simulink model "meat_1024pt_bee2_fpv2"  (Simulink 6.2)
settings: Solver=ode45  StartTime=0.0  StopTime=60000  RelTol=1e-3
undefined symbols (not defined in the file): BEE2_usr, bit_rev, pfb_coeff_gen_calc
libraries: xbsIndex_r3 x1085, casper_library x94, xps_library x27
(part 5 of 8)

== system meat_1024pt_bee2_fpv2/fft/fft_biplex0/biplex_core/fft_stage_1 ==
  in1 : Inport  Port=1  LatchInput=off
  in2 : Inport  Port=2  LatchInput=off
  sync : Inport  Port=3  LatchInput=off
  shift : Inport  Port=4  LatchInput=off
  Counter : xbsIndex_r3/Counter  cnt_type=Free Running  n_bits=FFTSize-FFTStage+1  bin_pt=0  arith_type=Unsigned  start_count=0  cnt_to=Inf  cnt_by_val=1  operation=Up  explicit_period=off  period=1  load_pin=off  rst=on  en=off  dbl_ovrd=off  show_param=off  use_rpm=off  gen_core=on
      settings: xl_area=[0, 0, 0, 0, 0, 0, 0]
  Delay : xbsIndex_r3/Delay  latency=1  reg_retiming=off  explicit_period=off  period=1  en=off  accept_only_valid=off  init_zero=on  dbl_ovrd=off  show_param=off
      settings: xl_area=[0, 0, 0, 0, 0, 0, 0]
  Mux : xbsIndex_r3/Mux  inputs=2  precision=Full  arith_type="Signed  (2's comp)"  n_bits=8  bin_pt=2  quantization=Truncate  overflow=Wrap  latency=1  explicit_period=off  period=1  en=off  dbl_ovrd=off  show_param=off  mux_type=off  use_rpm=off  gen_core=on
      settings: xl_area=[0, 0, 0, 0, 0, 0, 0]
  Mux1 : xbsIndex_r3/Mux  inputs=2  precision=Full  arith_type="Signed  (2's comp)"  n_bits=8  bin_pt=2  quantization=Truncate  overflow=Wrap  latency=1  explicit_period=off  period=1  en=off  dbl_ovrd=off  show_param=off  mux_type=off  use_rpm=off  gen_core=on
      settings: xl_area=[0, 0, 0, 0, 0, 0, 0]
  Slice : xbsIndex_r3/Slice  Orientation=up  mode=Lower Bit Location + Width  nbits=1  bit1=-(FFTStage - 1)  base1=MSB of Input  bit0=FFTStage - 1  base0=LSB of Input  boolean_output=on  explicit_period=off  period=1  dbl_ovrd=off
  Slice1 : xbsIndex_r3/Slice  mode=Upper Bit Location + Width  nbits=1  bit1=0  base1=MSB of Input  bit0=0  base0=LSB of Input  boolean_output=off  explicit_period=off  period=1  dbl_ovrd=off
  butterfly : Subsystem
  delay_b : Subsystem  BlockChoice=delay_bram
      link override delay_bram: bram_latency=bram_latency  DelayLen=2^(FFTSize-FFTStage)
      link override delay_bram/Constant2: equ=P=C
      link override delay_slr: DelayLen=2^(FFTSize-FFTStage)
      settings: AttributesFormatString=%<BlockChoice>  TemplateBlock=casper_library/Delays/delay  MemberBlocks=delay_bram,delay_slr
  delay_f : Subsystem  BlockChoice=delay_bram
      link override delay_bram: bram_latency=bram_latency  DelayLen=2^(FFTSize-FFTStage)
      link override delay_bram/Constant2: equ=P=C
      link override delay_slr: DelayLen=2^(FFTSize-FFTStage)
      settings: AttributesFormatString=%<BlockChoice>  TemplateBlock=casper_library/Delays/delay  MemberBlocks=delay_bram,delay_slr
  sync_delay : casper_library/Delays/sync_delay  DelayLen=2^(FFTSize - FFTStage)
      link override Constant: equ=P=C
      link override Constant1: equ=P=C
      link override Constant2: equ=P=C
      link override Constant3: equ=P=C
  out1 : Outport
  out2 : Outport  Port=2
  of : Outport  Port=3
  sync_out : Outport  Port=4
  wires:
  shift/1 -> Slice/1
  Delay/1 -> sync_delay/1
  sync/1 -> Counter/1, Delay/1
  Counter/1 -> Slice1/1
  Mux/1 -> butterfly/2(b)
  Mux1/1 -> delay_b/1(In1)
  delay_f/1(Out1) -> Mux1/3, Mux/2
  in1/1 -> Mux/3, Mux1/2
  Slice1/1 -> Mux/1, Mux1/1
  in2/1 -> delay_f/1(In1)
  delay_b/1(Out1) -> butterfly/1(a)
  sync_delay/1 -> butterfly/3(sync)
  Slice/1 -> butterfly/4(shift)
  butterfly/3(of) -> of/1
  butterfly/2(a-bw) -> out2/1
  butterfly/1(a+bw) -> out1/1
  butterfly/4(sync_out) -> sync_out/1

== system meat_1024pt_bee2_fpv2/fft/fft_biplex0/biplex_core/fft_stage_10 ==
  in1 : Inport  Port=1  LatchInput=off
  in2 : Inport  Port=2  LatchInput=off
  of_in : Inport  Port=3  LatchInput=off
  sync : Inport  Port=4  LatchInput=off
  shift : Inport  Port=5  LatchInput=off
  Counter : xbsIndex_r3/Counter  cnt_type=Free Running  n_bits=FFTSize-FFTStage+1  bin_pt=0  arith_type=Unsigned  start_count=0  cnt_to=Inf  cnt_by_val=1  operation=Up  explicit_period=off  period=1  load_pin=off  rst=on  en=off  dbl_ovrd=off  show_param=off  use_rpm=off  gen_core=on
      settings: xl_area=[0, 0, 0, 0, 0, 0, 0]
  Delay : xbsIndex_r3/Delay  latency=1  reg_retiming=off  explicit_period=off  period=1  en=off  accept_only_valid=off  init_zero=on  dbl_ovrd=off  show_param=off
      settings: xl_area=[0, 0, 0, 0, 0, 0, 0]
  Logical1 : xbsIndex_r3/Logical  logical_function=OR  inputs=2  precision=Full  arith_type=Unsigned  n_bits=8  bin_pt=2  align_bp=on  latency=1  explicit_period=on  period=1  en=off  dbl_ovrd=off  show_param=off
      settings: xl_area=[0, 0, 0, 0, 0, 0, 0]
  Mux : xbsIndex_r3/Mux  inputs=2  precision=Full  arith_type="Signed  (2's comp)"  n_bits=8  bin_pt=2  quantization=Truncate  overflow=Wrap  latency=1  explicit_period=off  period=1  en=off  dbl_ovrd=off  show_param=off  mux_type=off  use_rpm=off  gen_core=on
      settings: xl_area=[0, 0, 0, 0, 0, 0, 0]
  Mux1 : xbsIndex_r3/Mux  inputs=2  precision=Full  arith_type="Signed  (2's comp)"  n_bits=8  bin_pt=2  quantization=Truncate  overflow=Wrap  latency=1  explicit_period=off  period=1  en=off  dbl_ovrd=off  show_param=off  mux_type=off  use_rpm=off  gen_core=on
      settings: xl_area=[0, 0, 0, 0, 0, 0, 0]
  Slice : xbsIndex_r3/Slice  Orientation=up  mode=Lower Bit Location + Width  nbits=1  bit1=-(FFTStage - 1)  base1=MSB of Input  bit0=FFTStage - 1  base0=LSB of Input  boolean_output=on  explicit_period=off  period=1  dbl_ovrd=off
  Slice1 : xbsIndex_r3/Slice  mode=Upper Bit Location + Width  nbits=1  bit1=0  base1=MSB of Input  bit0=0  base0=LSB of Input  boolean_output=off  explicit_period=off  period=1  dbl_ovrd=off
  butterfly_direct : Subsystem  AncestorBlock=casper_library/FFTs/butterfly_direct  mask(butterfly_direct){FFTSize=10, Coeffs=getfield( getfield( get_param( gcb,'UserData'), 'parameters'),'Coeffs'), StepPeriod=0, BitWidth=18, add_latency=3, mult_latency=4, bram_latency=3, use_bram=0, quantization=Truncate, overflow=Wrap}
      mask prompts: FFTSize "Size of FFT: (2^?)"; Coeffs "Coefficients: (0 to 2^(FFTSize-1)-1)"; StepPeriod "Coefficient Step Period: (2^?)"; BitWidth "Output Bitwidth:"; add_latency "Add Latency"; mult_latency "Mult Latency"; bram_latency "BRAM Latency"; use_bram "Store Coefficients in BRAM"; quantization "Quantization Behavior"; overflow "Overflow Behavior"
      mask init:
      | butterfly_direct_init(gcb,...
      |               'FFTSize', FFTSize,...
      |               'Coeffs', Coeffs,...
      |               'StepPeriod', StepPeriod,...
      |               'BitWidth', BitWidth,...
      |               'add_latency', add_latency,...
      |               'mult_latency', mult_latency,...
      |               'bram_latency', bram_latency,...
      |               'use_bram',use_bram,...
      |               'quantization',quantization,...
      |               'overflow',overflow);
      settings: AttributesFormatString=|
      | FFTSize=10, Coeffs=[0    1    2    3    4    5    6    7    8    9   10   11   12   13   14   15   16   17   18   19   20   21   22   23   24   25   26   27   28   29   30   31   32   33   34   35   36   37   38   39   40   41   42   43   44   45   46   47   48   49   50   51   52   53   54   55   56   57   58   59   60   61   62   63   64   65   66   67   68   69   70   71   72   73   74   75   76   77   78   79   80   81   82   83   84   85   86   87   88   89   90   91   92   93   94   95   96   97   98   99  100  101  102  103  104  105  106  107  108  109  110  111  112  113  114  115  116  117  118  119  120  121  122  123  124  125  126  127  128  129  130  131  132  133  134  135  136  137  138  139  140  141  142  143  144  145  146  147  148  149  150  151  152  153  154  155  156  157  158  159  160  161  162  163  164  165  166  167  168  169  170  171  172  173  174  175  176  177  178  179  180  181  182  183  184  185  186  187  188  189  190  191  192  193  194  195  196  197  198  199  200  201  202  203  204  205  206  207  208  209  210  211  212  213  214  215  216  217  218  219  220  221  222  223  224  225  226  227  228  229  230  231  232  233  234  235  236  237  238  239  240  241  242  243  244  245  246  247  248  249  250  251  252  253  254  255  256  257  258  259  260  261  262  263  264  265  266  267  268  269  270  271  272  273  274  275  276  277  278  279  280  281  282  283  284  285  286  287  288  289  290  291  292  293  294  295  296  297  298  299  300  301  302  303  304  305  306  307  308  309  310  311  312  313  314  315  316  317  318  319  320  321  322  323  324  325  326  327  328  329  330  331  332  333  334  335  336  337  338  339  340  341  342  343  344  345  346  347  348  349  350  351  352  353  354  355  356  357  358  359  360  361  362  363  364  365  366  367  368  369  370  371  372  373  374  375  376  377  378  379  380  381  382  383  384  385  386  387  388  389  390  391  392  393  394  395  396  397  398  399  400  401  402  403  404  405  406  407  408  409  410  411  412  413  414  415  416  417  418  419  420  421  422  423  424  425  426  427  428  429  430  431  432  433  434  435  436  437  438  439  440  441  442  443  444  445  446  447  448  449  450  451  452  453  454  455  456  457  458  459  460  461  462  463  464  465  466  467  468  469  470  471  472  473  474  475  476  477  478  479  480  481  482  483  484  485  486  487  488  489  490  491  492  493  494  495  496  497  498  499  500  501  502  503  504  505  506  507  508  509  510  511],
      |  StepPeriod=0, BitWidth=18
      mask StyleString: edit,edit,edit,edit,edit,edit,edit,edit,popup(Truncate|Round  (unbiased: +/- Inf)|Round  (unbiased: Even Values)),popup(Wrap|Saturate|Error)
  delay_b : Subsystem  BlockChoice=delay_slr
      link override delay_bram: bram_latency=bram_latency  DelayLen=2^(FFTSize-FFTStage)
      link override delay_slr: DelayLen=2^(FFTSize-FFTStage)
      settings: AttributesFormatString=%<BlockChoice>  TemplateBlock=casper_library/Delays/delay  MemberBlocks=delay_bram,delay_slr
  delay_f : Subsystem  BlockChoice=delay_slr
      link override delay_bram: bram_latency=bram_latency  DelayLen=2^(FFTSize-FFTStage)
      link override delay_slr: DelayLen=2^(FFTSize-FFTStage)
      settings: AttributesFormatString=%<BlockChoice>  TemplateBlock=casper_library/Delays/delay  MemberBlocks=delay_bram,delay_slr
  sync_delay : casper_library/Delays/sync_delay  DelayLen=2^(FFTSize - FFTStage)
      link override Constant: equ=P=C
      link override Constant1: equ=P=C
      link override Constant2: equ=P=C
      link override Constant3: equ=P=C
  out1 : Outport
  out2 : Outport  Port=2
  of : Outport  Port=3
  sync_out : Outport  Port=4
  wires:
  butterfly_direct/4(sync_out) -> sync_out/1
  butterfly_direct/1(a+bw) -> out1/1
  butterfly_direct/2(a-bw) -> out2/1
  butterfly_direct/3(of) -> Logical1/1
  Slice/1 -> butterfly_direct/4(shift)
  sync_delay/1 -> butterfly_direct/3(sync)
  delay_b/1(Out1) -> butterfly_direct/1(a)
  in2/1 -> delay_f/1(In1)
  Slice1/1 -> Mux1/1, Mux/1
  in1/1 -> Mux1/2, Mux/3
  delay_f/1(Out1) -> Mux/2, Mux1/3
  Mux1/1 -> delay_b/1(In1)
  Mux/1 -> butterfly_direct/2(b)
  Counter/1 -> Slice1/1
  sync/1 -> Delay/1, Counter/1
  Delay/1 -> sync_delay/1
  Logical1/1 -> of/1
  of_in/1 -> Logical1/2
  shift/1 -> Slice/1

== system meat_1024pt_bee2_fpv2/fft/fft_biplex0/biplex_core/fft_stage_2 ==
  in1 : Inport  Port=1  LatchInput=off
  in2 : Inport  Port=2  LatchInput=off
  of_in : Inport  Port=3  LatchInput=off
  sync : Inport  Port=4  LatchInput=off
  shift : Inport  Port=5  LatchInput=off
  Counter : xbsIndex_r3/Counter  cnt_type=Free Running  n_bits=FFTSize-FFTStage+1  bin_pt=0  arith_type=Unsigned  start_count=0  cnt_to=Inf  cnt_by_val=1  operation=Up  explicit_period=off  period=1  load_pin=off  rst=on  en=off  dbl_ovrd=off  show_param=off  use_rpm=off  gen_core=on
      settings: xl_area=[0, 0, 0, 0, 0, 0, 0]
  Delay : xbsIndex_r3/Delay  latency=1  reg_retiming=off  explicit_period=off  period=1  en=off  accept_only_valid=off  init_zero=on  dbl_ovrd=off  show_param=off
      settings: xl_area=[0, 0, 0, 0, 0, 0, 0]
  Logical1 : xbsIndex_r3/Logical  logical_function=OR  inputs=2  precision=Full  arith_type=Unsigned  n_bits=8  bin_pt=2  align_bp=on  latency=1  explicit_period=on  period=1  en=off  dbl_ovrd=off  show_param=off
      settings: xl_area=[0, 0, 0, 0, 0, 0, 0]
  Mux : xbsIndex_r3/Mux  inputs=2  precision=Full  arith_type="Signed  (2's comp)"  n_bits=8  bin_pt=2  quantization=Truncate  overflow=Wrap  latency=1  explicit_period=off  period=1  en=off  dbl_ovrd=off  show_param=off  mux_type=off  use_rpm=off  gen_core=on
      settings: xl_area=[0, 0, 0, 0, 0, 0, 0]
  Mux1 : xbsIndex_r3/Mux  inputs=2  precision=Full  arith_type="Signed  (2's comp)"  n_bits=8  bin_pt=2  quantization=Truncate  overflow=Wrap  latency=1  explicit_period=off  period=1  en=off  dbl_ovrd=off  show_param=off  mux_type=off  use_rpm=off  gen_core=on
      settings: xl_area=[0, 0, 0, 0, 0, 0, 0]
  Slice : xbsIndex_r3/Slice  Orientation=up  mode=Lower Bit Location + Width  nbits=1  bit1=-(FFTStage - 1)  base1=MSB of Input  bit0=FFTStage - 1  base0=LSB of Input  boolean_output=on  explicit_period=off  period=1  dbl_ovrd=off
  Slice1 : xbsIndex_r3/Slice  mode=Upper Bit Location + Width  nbits=1  bit1=0  base1=MSB of Input  bit0=0  base0=LSB of Input  boolean_output=off  explicit_period=off  period=1  dbl_ovrd=off
  butterfly_direct : Subsystem  AncestorBlock=casper_library/FFTs/butterfly_direct  mask(butterfly_direct){FFTSize=10, Coeffs=[0 1], StepPeriod=8, BitWidth=18, add_latency=3, mult_latency=4, bram_latency=3, use_bram=1, quantization=Truncate, overflow=Wrap}
      mask prompts: FFTSize "Size of FFT: (2^?)"; Coeffs "Coefficients: (0 to 2^(FFTSize-1)-1)"; StepPeriod "Coefficient Step Period: (2^?)"; BitWidth "Output Bitwidth:"; add_latency "Add Latency"; mult_latency "Mult Latency"; bram_latency "BRAM Latency"; use_bram "Store Coefficients in BRAM"; quantization "Quantization Behavior"; overflow "Overflow Behavior"
      mask init: same as meat_1024pt_bee2_fpv2/fft/fft_biplex0/biplex_core/fft_stage_10/butterfly_direct
      settings: AttributesFormatString=|
      | FFTSize=10, Coeffs=[0  1],
      |  StepPeriod=8, BitWidth=18
      mask StyleString: edit,edit,edit,edit,edit,edit,edit,edit,popup(Truncate|Round  (unbiased: +/- Inf)|Round  (unbiased: Even Values)),popup(Wrap|Saturate|Error)
  delay_b : Subsystem  BlockChoice=delay_bram
      link override delay_bram: bram_latency=bram_latency  DelayLen=2^(FFTSize-FFTStage)
      link override delay_bram/Constant2: equ=P=C
      link override delay_slr: DelayLen=2^(FFTSize-FFTStage)
      settings: AttributesFormatString=%<BlockChoice>  TemplateBlock=casper_library/Delays/delay  MemberBlocks=delay_bram,delay_slr
  delay_f : Subsystem  BlockChoice=delay_bram
      link override delay_bram: bram_latency=bram_latency  DelayLen=2^(FFTSize-FFTStage)
      link override delay_bram/Constant2: equ=P=C
      link override delay_slr: DelayLen=2^(FFTSize-FFTStage)
      settings: AttributesFormatString=%<BlockChoice>  TemplateBlock=casper_library/Delays/delay  MemberBlocks=delay_bram,delay_slr
  sync_delay : casper_library/Delays/sync_delay  DelayLen=2^(FFTSize - FFTStage)
      link override Constant: equ=P=C
      link override Constant1: equ=P=C
      link override Constant2: equ=P=C
      link override Constant3: equ=P=C
  out1 : Outport
  out2 : Outport  Port=2
  of : Outport  Port=3
  sync_out : Outport  Port=4
  wires:
  butterfly_direct/4(sync_out) -> sync_out/1
  butterfly_direct/1(a+bw) -> out1/1
  butterfly_direct/2(a-bw) -> out2/1
  butterfly_direct/3(of) -> Logical1/1
  Slice/1 -> butterfly_direct/4(shift)
  sync_delay/1 -> butterfly_direct/3(sync)
  delay_b/1(Out1) -> butterfly_direct/1(a)
  in2/1 -> delay_f/1(In1)
  Slice1/1 -> Mux1/1, Mux/1
  in1/1 -> Mux1/2, Mux/3
  delay_f/1(Out1) -> Mux/2, Mux1/3
  Mux1/1 -> delay_b/1(In1)
  Mux/1 -> butterfly_direct/2(b)
  Counter/1 -> Slice1/1
  sync/1 -> Delay/1, Counter/1
  Delay/1 -> sync_delay/1
  Logical1/1 -> of/1
  of_in/1 -> Logical1/2
  shift/1 -> Slice/1

== system meat_1024pt_bee2_fpv2/fft/fft_biplex0/biplex_core/fft_stage_3 ==
  in1 : Inport  Port=1  LatchInput=off
  in2 : Inport  Port=2  LatchInput=off
  of_in : Inport  Port=3  LatchInput=off
  sync : Inport  Port=4  LatchInput=off
  shift : Inport  Port=5  LatchInput=off
  Counter : xbsIndex_r3/Counter  cnt_type=Free Running  n_bits=FFTSize-FFTStage+1  bin_pt=0  arith_type=Unsigned  start_count=0  cnt_to=Inf  cnt_by_val=1  operation=Up  explicit_period=off  period=1  load_pin=off  rst=on  en=off  dbl_ovrd=off  show_param=off  use_rpm=off  gen_core=on
      settings: xl_area=[0, 0, 0, 0, 0, 0, 0]
  Delay : xbsIndex_r3/Delay  latency=1  reg_retiming=off  explicit_period=off  period=1  en=off  accept_only_valid=off  init_zero=on  dbl_ovrd=off  show_param=off
      settings: xl_area=[0, 0, 0, 0, 0, 0, 0]
  Logical1 : xbsIndex_r3/Logical  logical_function=OR  inputs=2  precision=Full  arith_type=Unsigned  n_bits=8  bin_pt=2  align_bp=on  latency=1  explicit_period=on  period=1  en=off  dbl_ovrd=off  show_param=off
      settings: xl_area=[0, 0, 0, 0, 0, 0, 0]
  Mux : xbsIndex_r3/Mux  inputs=2  precision=Full  arith_type="Signed  (2's comp)"  n_bits=8  bin_pt=2  quantization=Truncate  overflow=Wrap  latency=1  explicit_period=off  period=1  en=off  dbl_ovrd=off  show_param=off  mux_type=off  use_rpm=off  gen_core=on
      settings: xl_area=[0, 0, 0, 0, 0, 0, 0]
  Mux1 : xbsIndex_r3/Mux  inputs=2  precision=Full  arith_type="Signed  (2's comp)"  n_bits=8  bin_pt=2  quantization=Truncate  overflow=Wrap  latency=1  explicit_period=off  period=1  en=off  dbl_ovrd=off  show_param=off  mux_type=off  use_rpm=off  gen_core=on
      settings: xl_area=[0, 0, 0, 0, 0, 0, 0]
  Slice : xbsIndex_r3/Slice  Orientation=up  mode=Lower Bit Location + Width  nbits=1  bit1=-(FFTStage - 1)  base1=MSB of Input  bit0=FFTStage - 1  base0=LSB of Input  boolean_output=on  explicit_period=off  period=1  dbl_ovrd=off
  Slice1 : xbsIndex_r3/Slice  mode=Upper Bit Location + Width  nbits=1  bit1=0  base1=MSB of Input  bit0=0  base0=LSB of Input  boolean_output=off  explicit_period=off  period=1  dbl_ovrd=off
  butterfly_direct : Subsystem  AncestorBlock=casper_library/FFTs/butterfly_direct  mask(butterfly_direct){FFTSize=10, Coeffs=[0 1 2 3], StepPeriod=7, BitWidth=18, add_latency=3, mult_latency=4, bram_latency=3, use_bram=1, quantization=Truncate, overflow=Wrap}
      mask prompts: FFTSize "Size of FFT: (2^?)"; Coeffs "Coefficients: (0 to 2^(FFTSize-1)-1)"; StepPeriod "Coefficient Step Period: (2^?)"; BitWidth "Output Bitwidth:"; add_latency "Add Latency"; mult_latency "Mult Latency"; bram_latency "BRAM Latency"; use_bram "Store Coefficients in BRAM"; quantization "Quantization Behavior"; overflow "Overflow Behavior"
      mask init: same as meat_1024pt_bee2_fpv2/fft/fft_biplex0/biplex_core/fft_stage_10/butterfly_direct
      settings: AttributesFormatString=|
      | FFTSize=10, Coeffs=[0  1  2  3],
      |  StepPeriod=7, BitWidth=18
      mask StyleString: edit,edit,edit,edit,edit,edit,edit,edit,popup(Truncate|Round  (unbiased: +/- Inf)|Round  (unbiased: Even Values)),popup(Wrap|Saturate|Error)
  delay_b : Subsystem  BlockChoice=delay_bram
      link override delay_bram: bram_latency=bram_latency  DelayLen=2^(FFTSize-FFTStage)
      link override delay_bram/Constant2: equ=P=C
      link override delay_slr: DelayLen=2^(FFTSize-FFTStage)
      settings: AttributesFormatString=%<BlockChoice>  TemplateBlock=casper_library/Delays/delay  MemberBlocks=delay_bram,delay_slr
  delay_f : Subsystem  BlockChoice=delay_bram
      link override delay_bram: bram_latency=bram_latency  DelayLen=2^(FFTSize-FFTStage)
      link override delay_bram/Constant2: equ=P=C
      link override delay_slr: DelayLen=2^(FFTSize-FFTStage)
      settings: AttributesFormatString=%<BlockChoice>  TemplateBlock=casper_library/Delays/delay  MemberBlocks=delay_bram,delay_slr
  sync_delay : casper_library/Delays/sync_delay  DelayLen=2^(FFTSize - FFTStage)
      link override Constant: equ=P=C
      link override Constant1: equ=P=C
      link override Constant2: equ=P=C
      link override Constant3: equ=P=C
  out1 : Outport
  out2 : Outport  Port=2
  of : Outport  Port=3
  sync_out : Outport  Port=4
  wires:
  butterfly_direct/4(sync_out) -> sync_out/1
  butterfly_direct/1(a+bw) -> out1/1
  butterfly_direct/2(a-bw) -> out2/1
  butterfly_direct/3(of) -> Logical1/1
  Slice/1 -> butterfly_direct/4(shift)
  sync_delay/1 -> butterfly_direct/3(sync)
  delay_b/1(Out1) -> butterfly_direct/1(a)
  in2/1 -> delay_f/1(In1)
  Slice1/1 -> Mux1/1, Mux/1
  in1/1 -> Mux1/2, Mux/3
  delay_f/1(Out1) -> Mux/2, Mux1/3
  Mux1/1 -> delay_b/1(In1)
  Mux/1 -> butterfly_direct/2(b)
  Counter/1 -> Slice1/1
  sync/1 -> Delay/1, Counter/1
  Delay/1 -> sync_delay/1
  Logical1/1 -> of/1
  of_in/1 -> Logical1/2
  shift/1 -> Slice/1

== system meat_1024pt_bee2_fpv2/fft/fft_biplex0/biplex_core/fft_stage_4 ==
  in1 : Inport  Port=1  LatchInput=off
  in2 : Inport  Port=2  LatchInput=off
  of_in : Inport  Port=3  LatchInput=off
  sync : Inport  Port=4  LatchInput=off
  shift : Inport  Port=5  LatchInput=off
  Counter : xbsIndex_r3/Counter  cnt_type=Free Running  n_bits=FFTSize-FFTStage+1  bin_pt=0  arith_type=Unsigned  start_count=0  cnt_to=Inf  cnt_by_val=1  operation=Up  explicit_period=off  period=1  load_pin=off  rst=on  en=off  dbl_ovrd=off  show_param=off  use_rpm=off  gen_core=on
      settings: xl_area=[0, 0, 0, 0, 0, 0, 0]
  Delay : xbsIndex_r3/Delay  latency=1  reg_retiming=off  explicit_period=off  period=1  en=off  accept_only_valid=off  init_zero=on  dbl_ovrd=off  show_param=off
      settings: xl_area=[0, 0, 0, 0, 0, 0, 0]
  Logical1 : xbsIndex_r3/Logical  logical_function=OR  inputs=2  precision=Full  arith_type=Unsigned  n_bits=8  bin_pt=2  align_bp=on  latency=1  explicit_period=on  period=1  en=off  dbl_ovrd=off  show_param=off
      settings: xl_area=[0, 0, 0, 0, 0, 0, 0]
  Mux : xbsIndex_r3/Mux  inputs=2  precision=Full  arith_type="Signed  (2's comp)"  n_bits=8  bin_pt=2  quantization=Truncate  overflow=Wrap  latency=1  explicit_period=off  period=1  en=off  dbl_ovrd=off  show_param=off  mux_type=off  use_rpm=off  gen_core=on
      settings: xl_area=[0, 0, 0, 0, 0, 0, 0]
  Mux1 : xbsIndex_r3/Mux  inputs=2  precision=Full  arith_type="Signed  (2's comp)"  n_bits=8  bin_pt=2  quantization=Truncate  overflow=Wrap  latency=1  explicit_period=off  period=1  en=off  dbl_ovrd=off  show_param=off  mux_type=off  use_rpm=off  gen_core=on
      settings: xl_area=[0, 0, 0, 0, 0, 0, 0]
  Slice : xbsIndex_r3/Slice  Orientation=up  mode=Lower Bit Location + Width  nbits=1  bit1=-(FFTStage - 1)  base1=MSB of Input  bit0=FFTStage - 1  base0=LSB of Input  boolean_output=on  explicit_period=off  period=1  dbl_ovrd=off
  Slice1 : xbsIndex_r3/Slice  mode=Upper Bit Location + Width  nbits=1  bit1=0  base1=MSB of Input  bit0=0  base0=LSB of Input  boolean_output=off  explicit_period=off  period=1  dbl_ovrd=off
  butterfly_direct : Subsystem  AncestorBlock=casper_library/FFTs/butterfly_direct  mask(butterfly_direct){FFTSize=10, Coeffs=[0 1 2 3 4 5 6 7], StepPeriod=6, BitWidth=18, add_latency=3, mult_latency=4, bram_latency=3, use_bram=1, quantization=Truncate, overflow=Wrap}
      mask prompts: FFTSize "Size of FFT: (2^?)"; Coeffs "Coefficients: (0 to 2^(FFTSize-1)-1)"; StepPeriod "Coefficient Step Period: (2^?)"; BitWidth "Output Bitwidth:"; add_latency "Add Latency"; mult_latency "Mult Latency"; bram_latency "BRAM Latency"; use_bram "Store Coefficients in BRAM"; quantization "Quantization Behavior"; overflow "Overflow Behavior"
      mask init: same as meat_1024pt_bee2_fpv2/fft/fft_biplex0/biplex_core/fft_stage_10/butterfly_direct
      settings: AttributesFormatString=|
      | FFTSize=10, Coeffs=[0  1  2  3  4  5  6  7],
      |  StepPeriod=6, BitWidth=18
      mask StyleString: edit,edit,edit,edit,edit,edit,edit,edit,popup(Truncate|Round  (unbiased: +/- Inf)|Round  (unbiased: Even Values)),popup(Wrap|Saturate|Error)
  delay_b : Subsystem  BlockChoice=delay_bram
      link override delay_bram: bram_latency=bram_latency  DelayLen=2^(FFTSize-FFTStage)
      link override delay_bram/Constant2: equ=P=C
      link override delay_slr: DelayLen=2^(FFTSize-FFTStage)
      settings: AttributesFormatString=%<BlockChoice>  TemplateBlock=casper_library/Delays/delay  MemberBlocks=delay_bram,delay_slr
  delay_f : Subsystem  BlockChoice=delay_bram
      link override delay_bram: bram_latency=bram_latency  DelayLen=2^(FFTSize-FFTStage)
      link override delay_bram/Constant2: equ=P=C
      link override delay_slr: DelayLen=2^(FFTSize-FFTStage)
      settings: AttributesFormatString=%<BlockChoice>  TemplateBlock=casper_library/Delays/delay  MemberBlocks=delay_bram,delay_slr
  sync_delay : casper_library/Delays/sync_delay  DelayLen=2^(FFTSize - FFTStage)
      link override Constant: equ=P=C
      link override Constant1: equ=P=C
      link override Constant2: equ=P=C
      link override Constant3: equ=P=C
  out1 : Outport
  out2 : Outport  Port=2
  of : Outport  Port=3
  sync_out : Outport  Port=4
  wires:
  butterfly_direct/4(sync_out) -> sync_out/1
  butterfly_direct/1(a+bw) -> out1/1
  butterfly_direct/2(a-bw) -> out2/1
  butterfly_direct/3(of) -> Logical1/1
  Slice/1 -> butterfly_direct/4(shift)
  sync_delay/1 -> butterfly_direct/3(sync)
  delay_b/1(Out1) -> butterfly_direct/1(a)
  in2/1 -> delay_f/1(In1)
  Slice1/1 -> Mux1/1, Mux/1
  in1/1 -> Mux1/2, Mux/3
  delay_f/1(Out1) -> Mux/2, Mux1/3
  Mux1/1 -> delay_b/1(In1)
  Mux/1 -> butterfly_direct/2(b)
  Counter/1 -> Slice1/1
  sync/1 -> Delay/1, Counter/1
  Delay/1 -> sync_delay/1
  Logical1/1 -> of/1
  of_in/1 -> Logical1/2
  shift/1 -> Slice/1

== system meat_1024pt_bee2_fpv2/fft/fft_biplex0/biplex_core/fft_stage_5 ==
  in1 : Inport  Port=1  LatchInput=off
  in2 : Inport  Port=2  LatchInput=off
  of_in : Inport  Port=3  LatchInput=off
  sync : Inport  Port=4  LatchInput=off
  shift : Inport  Port=5  LatchInput=off
  Counter : xbsIndex_r3/Counter  cnt_type=Free Running  n_bits=FFTSize-FFTStage+1  bin_pt=0  arith_type=Unsigned  start_count=0  cnt_to=Inf  cnt_by_val=1  operation=Up  explicit_period=off  period=1  load_pin=off  rst=on  en=off  dbl_ovrd=off  show_param=off  use_rpm=off  gen_core=on
      settings: xl_area=[0, 0, 0, 0, 0, 0, 0]
  Delay : xbsIndex_r3/Delay  latency=1  reg_retiming=off  explicit_period=off  period=1  en=off  accept_only_valid=off  init_zero=on  dbl_ovrd=off  show_param=off
      settings: xl_area=[0, 0, 0, 0, 0, 0, 0]
  Logical1 : xbsIndex_r3/Logical  logical_function=OR  inputs=2  precision=Full  arith_type=Unsigned  n_bits=8  bin_pt=2  align_bp=on  latency=1  explicit_period=on  period=1  en=off  dbl_ovrd=off  show_param=off
      settings: xl_area=[0, 0, 0, 0, 0, 0, 0]
  Mux : xbsIndex_r3/Mux  inputs=2  precision=Full  arith_type="Signed  (2's comp)"  n_bits=8  bin_pt=2  quantization=Truncate  overflow=Wrap  latency=1  explicit_period=off  period=1  en=off  dbl_ovrd=off  show_param=off  mux_type=off  use_rpm=off  gen_core=on
      settings: xl_area=[0, 0, 0, 0, 0, 0, 0]
  Mux1 : xbsIndex_r3/Mux  inputs=2  precision=Full  arith_type="Signed  (2's comp)"  n_bits=8  bin_pt=2  quantization=Truncate  overflow=Wrap  latency=1  explicit_period=off  period=1  en=off  dbl_ovrd=off  show_param=off  mux_type=off  use_rpm=off  gen_core=on
      settings: xl_area=[0, 0, 0, 0, 0, 0, 0]
  Slice : xbsIndex_r3/Slice  Orientation=up  mode=Lower Bit Location + Width  nbits=1  bit1=-(FFTStage - 1)  base1=MSB of Input  bit0=FFTStage - 1  base0=LSB of Input  boolean_output=on  explicit_period=off  period=1  dbl_ovrd=off
  Slice1 : xbsIndex_r3/Slice  mode=Upper Bit Location + Width  nbits=1  bit1=0  base1=MSB of Input  bit0=0  base0=LSB of Input  boolean_output=off  explicit_period=off  period=1  dbl_ovrd=off
  butterfly_direct : Subsystem  AncestorBlock=casper_library/FFTs/butterfly_direct  mask(butterfly_direct){FFTSize=10, Coeffs=[0 1 2 3 4 5 6 7 8 9 10 11 12 13 14 15], StepPeriod=5, BitWidth=18, add_latency=3, mult_latency=4, bram_latency=3, use_bram=0, quantization=Truncate, overflow=Wrap}
      mask prompts: FFTSize "Size of FFT: (2^?)"; Coeffs "Coefficients: (0 to 2^(FFTSize-1)-1)"; StepPeriod "Coefficient Step Period: (2^?)"; BitWidth "Output Bitwidth:"; add_latency "Add Latency"; mult_latency "Mult Latency"; bram_latency "BRAM Latency"; use_bram "Store Coefficients in BRAM"; quantization "Quantization Behavior"; overflow "Overflow Behavior"
      mask init: same as meat_1024pt_bee2_fpv2/fft/fft_biplex0/biplex_core/fft_stage_10/butterfly_direct
      settings: AttributesFormatString=|
      | FFTSize=10, Coeffs=[0   1   2   3   4   5   6   7   8   9  10  11  12  13  14  15],
      |  StepPeriod=5, BitWidth=18
      mask StyleString: edit,edit,edit,edit,edit,edit,edit,edit,popup(Truncate|Round  (unbiased: +/- Inf)|Round  (unbiased: Even Values)),popup(Wrap|Saturate|Error)
  delay_b : Subsystem  BlockChoice=delay_slr
      link override delay_bram: bram_latency=bram_latency  DelayLen=2^(FFTSize-FFTStage)
      link override delay_bram/Constant2: equ=P=C
      link override delay_slr: DelayLen=2^(FFTSize-FFTStage)
      settings: AttributesFormatString=%<BlockChoice>  TemplateBlock=casper_library/Delays/delay  MemberBlocks=delay_bram,delay_slr
  delay_f : Subsystem  BlockChoice=delay_slr
      link override delay_bram: bram_latency=bram_latency  DelayLen=2^(FFTSize-FFTStage)
      link override delay_bram/Constant2: equ=P=C
      link override delay_slr: DelayLen=2^(FFTSize-FFTStage)
      settings: AttributesFormatString=%<BlockChoice>  TemplateBlock=casper_library/Delays/delay  MemberBlocks=delay_bram,delay_slr
  sync_delay : casper_library/Delays/sync_delay  DelayLen=2^(FFTSize - FFTStage)
      link override Constant: equ=P=C
      link override Constant1: equ=P=C
      link override Constant2: equ=P=C
      link override Constant3: equ=P=C
  out1 : Outport
  out2 : Outport  Port=2
  of : Outport  Port=3
  sync_out : Outport  Port=4
  wires:
  butterfly_direct/4(sync_out) -> sync_out/1
  butterfly_direct/1(a+bw) -> out1/1
  butterfly_direct/2(a-bw) -> out2/1
  butterfly_direct/3(of) -> Logical1/1
  Slice/1 -> butterfly_direct/4(shift)
  sync_delay/1 -> butterfly_direct/3(sync)
  delay_b/1(Out1) -> butterfly_direct/1(a)
  in2/1 -> delay_f/1(In1)
  Slice1/1 -> Mux1/1, Mux/1
  in1/1 -> Mux1/2, Mux/3
  delay_f/1(Out1) -> Mux/2, Mux1/3
  Mux1/1 -> delay_b/1(In1)
  Mux/1 -> butterfly_direct/2(b)
  Counter/1 -> Slice1/1
  sync/1 -> Delay/1, Counter/1
  Delay/1 -> sync_delay/1
  Logical1/1 -> of/1
  of_in/1 -> Logical1/2
  shift/1 -> Slice/1

== system meat_1024pt_bee2_fpv2/fft/fft_biplex0/biplex_core/fft_stage_6 ==
  in1 : Inport  Port=1  LatchInput=off
  in2 : Inport  Port=2  LatchInput=off
  of_in : Inport  Port=3  LatchInput=off
  sync : Inport  Port=4  LatchInput=off
  shift : Inport  Port=5  LatchInput=off
  Counter : xbsIndex_r3/Counter  cnt_type=Free Running  n_bits=FFTSize-FFTStage+1  bin_pt=0  arith_type=Unsigned  start_count=0  cnt_to=Inf  cnt_by_val=1  operation=Up  explicit_period=off  period=1  load_pin=off  rst=on  en=off  dbl_ovrd=off  show_param=off  use_rpm=off  gen_core=on
      settings: xl_area=[0, 0, 0, 0, 0, 0, 0]
  Delay : xbsIndex_r3/Delay  latency=1  reg_retiming=off  explicit_period=off  period=1  en=off  accept_only_valid=off  init_zero=on  dbl_ovrd=off  show_param=off
      settings: xl_area=[0, 0, 0, 0, 0, 0, 0]
  Logical1 : xbsIndex_r3/Logical  logical_function=OR  inputs=2  precision=Full  arith_type=Unsigned  n_bits=8  bin_pt=2  align_bp=on  latency=1  explicit_period=on  period=1  en=off  dbl_ovrd=off  show_param=off
      settings: xl_area=[0, 0, 0, 0, 0, 0, 0]
  Mux : xbsIndex_r3/Mux  inputs=2  precision=Full  arith_type="Signed  (2's comp)"  n_bits=8  bin_pt=2  quantization=Truncate  overflow=Wrap  latency=1  explicit_period=off  period=1  en=off  dbl_ovrd=off  show_param=off  mux_type=off  use_rpm=off  gen_core=on
      settings: xl_area=[0, 0, 0, 0, 0, 0, 0]
  Mux1 : xbsIndex_r3/Mux  inputs=2  precision=Full  arith_type="Signed  (2's comp)"  n_bits=8  bin_pt=2  quantization=Truncate  overflow=Wrap  latency=1  explicit_period=off  period=1  en=off  dbl_ovrd=off  show_param=off  mux_type=off  use_rpm=off  gen_core=on
      settings: xl_area=[0, 0, 0, 0, 0, 0, 0]
  Slice : xbsIndex_r3/Slice  Orientation=up  mode=Lower Bit Location + Width  nbits=1  bit1=-(FFTStage - 1)  base1=MSB of Input  bit0=FFTStage - 1  base0=LSB of Input  boolean_output=on  explicit_period=off  period=1  dbl_ovrd=off
  Slice1 : xbsIndex_r3/Slice  mode=Upper Bit Location + Width  nbits=1  bit1=0  base1=MSB of Input  bit0=0  base0=LSB of Input  boolean_output=off  explicit_period=off  period=1  dbl_ovrd=off
  butterfly_direct : Subsystem  AncestorBlock=casper_library/FFTs/butterfly_direct  mask(butterfly_direct){FFTSize=10, Coeffs=[0 1 2 3 4 5 6 7 8 9 10 11 12 13 14 15 16 17 18 19 20 21 22 23 24 25 26 27 28 29 30 31], StepPeriod=4, BitWidth=18, add_latency=3, mult_latency=4, bram_latency=3, use_bram=0, quantization=Truncate, overflow=Wrap}
      mask prompts: FFTSize "Size of FFT: (2^?)"; Coeffs "Coefficients: (0 to 2^(FFTSize-1)-1)"; StepPeriod "Coefficient Step Period: (2^?)"; BitWidth "Output Bitwidth:"; add_latency "Add Latency"; mult_latency "Mult Latency"; bram_latency "BRAM Latency"; use_bram "Store Coefficients in BRAM"; quantization "Quantization Behavior"; overflow "Overflow Behavior"
      mask init: same as meat_1024pt_bee2_fpv2/fft/fft_biplex0/biplex_core/fft_stage_10/butterfly_direct
      settings: AttributesFormatString=|
      | FFTSize=10, Coeffs=[0   1   2   3   4   5   6   7   8   9  10  11  12  13  14  15  16  17  18  19  20  21  22  23  24  25  26  27  28  29  30  31],
      |  StepPeriod=4, BitWidth=18
      mask StyleString: edit,edit,edit,edit,edit,edit,edit,edit,popup(Truncate|Round  (unbiased: +/- Inf)|Round  (unbiased: Even Values)),popup(Wrap|Saturate|Error)
  delay_b : Subsystem  BlockChoice=delay_slr
      link override delay_bram: bram_latency=bram_latency  DelayLen=2^(FFTSize-FFTStage)
      link override delay_slr: DelayLen=2^(FFTSize-FFTStage)
      settings: AttributesFormatString=%<BlockChoice>  TemplateBlock=casper_library/Delays/delay  MemberBlocks=delay_bram,delay_slr
  delay_f : Subsystem  BlockChoice=delay_slr
      link override delay_bram: bram_latency=bram_latency  DelayLen=2^(FFTSize-FFTStage)
      link override delay_slr: DelayLen=2^(FFTSize-FFTStage)
      settings: AttributesFormatString=%<BlockChoice>  TemplateBlock=casper_library/Delays/delay  MemberBlocks=delay_bram,delay_slr
  sync_delay : casper_library/Delays/sync_delay  DelayLen=2^(FFTSize - FFTStage)
      link override Constant: equ=P=C
      link override Constant1: equ=P=C
      link override Constant2: equ=P=C
      link override Constant3: equ=P=C
  out1 : Outport
  out2 : Outport  Port=2
  of : Outport  Port=3
  sync_out : Outport  Port=4
  wires:
  butterfly_direct/4(sync_out) -> sync_out/1
  butterfly_direct/1(a+bw) -> out1/1
  butterfly_direct/2(a-bw) -> out2/1
  butterfly_direct/3(of) -> Logical1/1
  Slice/1 -> butterfly_direct/4(shift)
  sync_delay/1 -> butterfly_direct/3(sync)
  delay_b/1(Out1) -> butterfly_direct/1(a)
  in2/1 -> delay_f/1(In1)
  Slice1/1 -> Mux1/1, Mux/1
  in1/1 -> Mux1/2, Mux/3
  delay_f/1(Out1) -> Mux/2, Mux1/3
  Mux1/1 -> delay_b/1(In1)
  Mux/1 -> butterfly_direct/2(b)
  Counter/1 -> Slice1/1
  sync/1 -> Delay/1, Counter/1
  Delay/1 -> sync_delay/1
  Logical1/1 -> of/1
  of_in/1 -> Logical1/2
  shift/1 -> Slice/1

== system meat_1024pt_bee2_fpv2/fft/fft_biplex0/biplex_core/fft_stage_7 ==
  in1 : Inport  Port=1  LatchInput=off
  in2 : Inport  Port=2  LatchInput=off
  of_in : Inport  Port=3  LatchInput=off
  sync : Inport  Port=4  LatchInput=off
  shift : Inport  Port=5  LatchInput=off
  Counter : xbsIndex_r3/Counter  cnt_type=Free Running  n_bits=FFTSize-FFTStage+1  bin_pt=0  arith_type=Unsigned  start_count=0  cnt_to=Inf  cnt_by_val=1  operation=Up  explicit_period=off  period=1  load_pin=off  rst=on  en=off  dbl_ovrd=off  show_param=off  use_rpm=off  gen_core=on
      settings: xl_area=[0, 0, 0, 0, 0, 0, 0]
  Delay : xbsIndex_r3/Delay  latency=1  reg_retiming=off  explicit_period=off  period=1  en=off  accept_only_valid=off  init_zero=on  dbl_ovrd=off  show_param=off
      settings: xl_area=[0, 0, 0, 0, 0, 0, 0]
  Logical1 : xbsIndex_r3/Logical  logical_function=OR  inputs=2  precision=Full  arith_type=Unsigned  n_bits=8  bin_pt=2  align_bp=on  latency=1  explicit_period=on  period=1  en=off  dbl_ovrd=off  show_param=off
      settings: xl_area=[0, 0, 0, 0, 0, 0, 0]
  Mux : xbsIndex_r3/Mux  inputs=2  precision=Full  arith_type="Signed  (2's comp)"  n_bits=8  bin_pt=2  quantization=Truncate  overflow=Wrap  latency=1  explicit_period=off  period=1  en=off  dbl_ovrd=off  show_param=off  mux_type=off  use_rpm=off  gen_core=on
      settings: xl_area=[0, 0, 0, 0, 0, 0, 0]
  Mux1 : xbsIndex_r3/Mux  inputs=2  precision=Full  arith_type="Signed  (2's comp)"  n_bits=8  bin_pt=2  quantization=Truncate  overflow=Wrap  latency=1  explicit_period=off  period=1  en=off  dbl_ovrd=off  show_param=off  mux_type=off  use_rpm=off  gen_core=on
      settings: xl_area=[0, 0, 0, 0, 0, 0, 0]
  Slice : xbsIndex_r3/Slice  Orientation=up  mode=Lower Bit Location + Width  nbits=1  bit1=-(FFTStage - 1)  base1=MSB of Input  bit0=FFTStage - 1  base0=LSB of Input  boolean_output=on  explicit_period=off  period=1  dbl_ovrd=off
  Slice1 : xbsIndex_r3/Slice  mode=Upper Bit Location + Width  nbits=1  bit1=0  base1=MSB of Input  bit0=0  base0=LSB of Input  boolean_output=off  explicit_period=off  period=1  dbl_ovrd=off
  butterfly_direct : Subsystem  AncestorBlock=casper_library/FFTs/butterfly_direct  mask(butterfly_direct){FFTSize=10, Coeffs=getfield( getfield( get_param( gcb,'UserData'), 'parameters'),'Coeffs'), StepPeriod=3, BitWidth=18, add_latency=3, mult_latency=4, bram_latency=3, use_bram=0, quantization=Truncate, overflow=Wrap}
      mask prompts: FFTSize "Size of FFT: (2^?)"; Coeffs "Coefficients: (0 to 2^(FFTSize-1)-1)"; StepPeriod "Coefficient Step Period: (2^?)"; BitWidth "Output Bitwidth:"; add_latency "Add Latency"; mult_latency "Mult Latency"; bram_latency "BRAM Latency"; use_bram "Store Coefficients in BRAM"; quantization "Quantization Behavior"; overflow "Overflow Behavior"
      mask init: same as meat_1024pt_bee2_fpv2/fft/fft_biplex0/biplex_core/fft_stage_10/butterfly_direct
      settings: AttributesFormatString=|
      | FFTSize=10, Coeffs=[0   1   2   3   4   5   6   7   8   9  10  11  12  13  14  15  16  17  18  19  20  21  22  23  24  25  26  27  28  29  30  31  32  33  34  35  36  37  38  39  40  41  42  43  44  45  46  47  48  49  50  51  52  53  54  55  56  57  58  59  60  61  62  63],
      |  StepPeriod=3, BitWidth=18
      mask StyleString: edit,edit,edit,edit,edit,edit,edit,edit,popup(Truncate|Round  (unbiased: +/- Inf)|Round  (unbiased: Even Values)),popup(Wrap|Saturate|Error)
  delay_b : Subsystem  BlockChoice=delay_slr
      link override delay_bram: bram_latency=bram_latency  DelayLen=2^(FFTSize-FFTStage)
      link override delay_slr: DelayLen=2^(FFTSize-FFTStage)
      settings: AttributesFormatString=%<BlockChoice>  TemplateBlock=casper_library/Delays/delay  MemberBlocks=delay_bram,delay_slr
  delay_f : Subsystem  BlockChoice=delay_slr
      link override delay_bram: bram_latency=bram_latency  DelayLen=2^(FFTSize-FFTStage)
      link override delay_slr: DelayLen=2^(FFTSize-FFTStage)
      settings: AttributesFormatString=%<BlockChoice>  TemplateBlock=casper_library/Delays/delay  MemberBlocks=delay_bram,delay_slr
  sync_delay : casper_library/Delays/sync_delay  DelayLen=2^(FFTSize - FFTStage)
      link override Constant: equ=P=C
      link override Constant1: equ=P=C
      link override Constant2: equ=P=C
      link override Constant3: equ=P=C
  out1 : Outport
  out2 : Outport  Port=2
  of : Outport  Port=3
  sync_out : Outport  Port=4
  wires:
  butterfly_direct/4(sync_out) -> sync_out/1
  butterfly_direct/1(a+bw) -> out1/1
  butterfly_direct/2(a-bw) -> out2/1
  butterfly_direct/3(of) -> Logical1/1
  Slice/1 -> butterfly_direct/4(shift)
  sync_delay/1 -> butterfly_direct/3(sync)
  delay_b/1(Out1) -> butterfly_direct/1(a)
  in2/1 -> delay_f/1(In1)
  Slice1/1 -> Mux1/1, Mux/1
  in1/1 -> Mux1/2, Mux/3
  delay_f/1(Out1) -> Mux/2, Mux1/3
  Mux1/1 -> delay_b/1(In1)
  Mux/1 -> butterfly_direct/2(b)
  Counter/1 -> Slice1/1
  sync/1 -> Delay/1, Counter/1
  Delay/1 -> sync_delay/1
  Logical1/1 -> of/1
  of_in/1 -> Logical1/2
  shift/1 -> Slice/1

== system meat_1024pt_bee2_fpv2/fft/fft_biplex0/biplex_core/fft_stage_8 ==
  in1 : Inport  Port=1  LatchInput=off
  in2 : Inport  Port=2  LatchInput=off
  of_in : Inport  Port=3  LatchInput=off
  sync : Inport  Port=4  LatchInput=off
  shift : Inport  Port=5  LatchInput=off
  Counter : xbsIndex_r3/Counter  cnt_type=Free Running  n_bits=FFTSize-FFTStage+1  bin_pt=0  arith_type=Unsigned  start_count=0  cnt_to=Inf  cnt_by_val=1  operation=Up  explicit_period=off  period=1  load_pin=off  rst=on  en=off  dbl_ovrd=off  show_param=off  use_rpm=off  gen_core=on
      settings: xl_area=[0, 0, 0, 0, 0, 0, 0]
  Delay : xbsIndex_r3/Delay  latency=1  reg_retiming=off  explicit_period=off  period=1  en=off  accept_only_valid=off  init_zero=on  dbl_ovrd=off  show_param=off
      settings: xl_area=[0, 0, 0, 0, 0, 0, 0]
  Logical1 : xbsIndex_r3/Logical  logical_function=OR  inputs=2  precision=Full  arith_type=Unsigned  n_bits=8  bin_pt=2  align_bp=on  latency=1  explicit_period=on  period=1  en=off  dbl_ovrd=off  show_param=off
      settings: xl_area=[0, 0, 0, 0, 0, 0, 0]
  Mux : xbsIndex_r3/Mux  inputs=2  precision=Full  arith_type="Signed  (2's comp)"  n_bits=8  bin_pt=2  quantization=Truncate  overflow=Wrap  latency=1  explicit_period=off  period=1  en=off  dbl_ovrd=off  show_param=off  mux_type=off  use_rpm=off  gen_core=on
      settings: xl_area=[0, 0, 0, 0, 0, 0, 0]
  Mux1 : xbsIndex_r3/Mux  inputs=2  precision=Full  arith_type="Signed  (2's comp)"  n_bits=8  bin_pt=2  quantization=Truncate  overflow=Wrap  latency=1  explicit_period=off  period=1  en=off  dbl_ovrd=off  show_param=off  mux_type=off  use_rpm=off  gen_core=on
      settings: xl_area=[0, 0, 0, 0, 0, 0, 0]
  Slice : xbsIndex_r3/Slice  Orientation=up  mode=Lower Bit Location + Width  nbits=1  bit1=-(FFTStage - 1)  base1=MSB of Input  bit0=FFTStage - 1  base0=LSB of Input  boolean_output=on  explicit_period=off  period=1  dbl_ovrd=off
  Slice1 : xbsIndex_r3/Slice  mode=Upper Bit Location + Width  nbits=1  bit1=0  base1=MSB of Input  bit0=0  base0=LSB of Input  boolean_output=off  explicit_period=off  period=1  dbl_ovrd=off
  butterfly_direct : Subsystem  AncestorBlock=casper_library/FFTs/butterfly_direct  mask(butterfly_direct){FFTSize=10, Coeffs=getfield( getfield( get_param( gcb,'UserData'), 'parameters'),'Coeffs'), StepPeriod=2, BitWidth=18, add_latency=3, mult_latency=4, bram_latency=3, use_bram=0, quantization=Truncate, overflow=Wrap}
      mask prompts: FFTSize "Size of FFT: (2^?)"; Coeffs "Coefficients: (0 to 2^(FFTSize-1)-1)"; StepPeriod "Coefficient Step Period: (2^?)"; BitWidth "Output Bitwidth:"; add_latency "Add Latency"; mult_latency "Mult Latency"; bram_latency "BRAM Latency"; use_bram "Store Coefficients in BRAM"; quantization "Quantization Behavior"; overflow "Overflow Behavior"
      mask init: same as meat_1024pt_bee2_fpv2/fft/fft_biplex0/biplex_core/fft_stage_10/butterfly_direct
      settings: AttributesFormatString=|
      | FFTSize=10, Coeffs=[0    1    2    3    4    5    6    7    8    9   10   11   12   13   14   15   16   17   18   19   20   21   22   23   24   25   26   27   28   29   30   31   32   33   34   35   36   37   38   39   40   41   42   43   44   45   46   47   48   49   50   51   52   53   54   55   56   57   58   59   60   61   62   63   64   65   66   67   68   69   70   71   72   73   74   75   76   77   78   79   80   81   82   83   84   85   86   87   88   89   90   91   92   93   94   95   96   97   98   99  100  101  102  103  104  105  106  107  108  109  110  111  112  113  114  115  116  117  118  119  120  121  122  123  124  125  126  127],
      |  StepPeriod=2, BitWidth=18
      mask StyleString: edit,edit,edit,edit,edit,edit,edit,edit,popup(Truncate|Round  (unbiased: +/- Inf)|Round  (unbiased: Even Values)),popup(Wrap|Saturate|Error)
  delay_b : Subsystem  BlockChoice=delay_slr
      link override delay_bram: bram_latency=bram_latency  DelayLen=2^(FFTSize-FFTStage)
      link override delay_slr: DelayLen=2^(FFTSize-FFTStage)
      settings: AttributesFormatString=%<BlockChoice>  TemplateBlock=casper_library/Delays/delay  MemberBlocks=delay_bram,delay_slr
  delay_f : Subsystem  BlockChoice=delay_slr
      link override delay_bram: bram_latency=bram_latency  DelayLen=2^(FFTSize-FFTStage)
      link override delay_slr: DelayLen=2^(FFTSize-FFTStage)
      settings: AttributesFormatString=%<BlockChoice>  TemplateBlock=casper_library/Delays/delay  MemberBlocks=delay_bram,delay_slr
  sync_delay : casper_library/Delays/sync_delay  DelayLen=2^(FFTSize - FFTStage)
      link override Constant: equ=P=C
      link override Constant1: equ=P=C
      link override Constant2: equ=P=C
      link override Constant3: equ=P=C
  out1 : Outport
  out2 : Outport  Port=2
  of : Outport  Port=3
  sync_out : Outport  Port=4
  wires:
  butterfly_direct/4(sync_out) -> sync_out/1
  butterfly_direct/1(a+bw) -> out1/1
  butterfly_direct/2(a-bw) -> out2/1
  butterfly_direct/3(of) -> Logical1/1
  Slice/1 -> butterfly_direct/4(shift)
  sync_delay/1 -> butterfly_direct/3(sync)
  delay_b/1(Out1) -> butterfly_direct/1(a)
  in2/1 -> delay_f/1(In1)
  Slice1/1 -> Mux1/1, Mux/1
  in1/1 -> Mux1/2, Mux/3
  delay_f/1(Out1) -> Mux/2, Mux1/3
  Mux1/1 -> delay_b/1(In1)
  Mux/1 -> butterfly_direct/2(b)
  Counter/1 -> Slice1/1
  sync/1 -> Delay/1, Counter/1
  Delay/1 -> sync_delay/1
  Logical1/1 -> of/1
  of_in/1 -> Logical1/2
  shift/1 -> Slice/1
